simulink model "EOP_harness"  (Simulink 7.7)
settings: Solver=FixedStepDiscrete  SolverMode=SingleTasking  StartTime=0.0  StopTime=100  FixedStep=0.1  RelTol=1e-3
InitFcn:
  | CD_EOP_DEBOUNCE_OORH.DataType = 'uin16';
  | CD_EOP_DEBOUNCE_OORH = 10;
  | 
  | CD_EOP_DEBOUNCE_OORL.DataType = 'uin16';
  | CD_EOP_DEBOUNCE_OORL = 10;
  | 
  | 
  | 
  | if signalbuilder('EOP_harness/Signal_Builder','activegroup') == 1
  |   CD_EOP_FUNCTION.DataType = 'uint8';
  |   CD_EOP_FUNCTION.Value = 255;
  | elseif signalbuilder('EOP_harness/Signal_Builder','activegroup') == 7
  |   CD_EOP_FUNCTION.DataType = 'uint8';
  |   CD_EOP_FUNCTION.Value = 1;
  | elseif signalbuilder('EOP_harness/Signal_Builder','activegroup') == 8
  |   CD_EOP_FUNCTION.DataType = 'uint8';
  |   CD_EOP_FUNCTION.Value = 1;
  | elseif signalbuilder('EOP_harness/Signal_Builder','activegroup') == 3
  |   CD_EOP_FUNCTION.DataType = 'uint8';
  |   CD_EOP_FUNCTION.Value = 2;
  | else
  |   CD_EOP_FUNCTION.DataType = 'uint8';
  |   CD_EOP_FUNCTION.Value = 0;
  | end
  | 
  | 
  | if signalbuilder('EOP_harness/Signal_Builder','activegroup') == 4
  |   CD_EOP_FAULT_DETECTION_FUNCTION.DataType = 'uint8';
  |   CD_EOP_FAULT_DETECTION_FUNCTION.Value = 0;
  | end
  | 
  | if signalbuilder('EOP_harness/Signal_Builder','activegroup') == 5
  |   CD_SHUTDOWN_FUNCTION.DataType = 'uint8';
  |   CD_SHUTDOWN_FUNCTION.Value = 255;
  | elseif signalbuilder('EOP_harness/Signal_Builder','activegroup') == 8
  |   CD_SHUTDOWN_FUNCTION.DataType = 'uint8';
  |   CD_SHUTDOWN_FUNCTION.Value = 255;
  | else
  |   CD_SHUTDOWN_FUNCTION.DataType = 'uint8';
  |   CD_SHUTDOWN_FUNCTION.Value = 0;
  | end
  | 
  | if signalbuilder('EOP_harness/Signal_Builder','activegroup') == 12
  |   CD_ECU_FUNCTION.DataType = 'uint8';
  |   CD_ECU_FUNCTION.Value = 0;
  | else
  |   CD_ECU_FUNCTION.DataType = 'uint8';
  |   CD_ECU_FUNCTION.Value = 255;
  | end
undefined symbols (not defined in the file): CD_EOP_DEBOUNCE_EXTREMELY_LOW, CD_EOP_DEBOUNCE_NORMAL, CD_EOP_DEBOUNCE_SHUTDOWN, CD_EOP_FILTER_VALUE, CD_EOP_SWITCH_LOW, ENGINE_RUNNING, EXTREMELY_LOW, INIT_NORMAL, MXGTW_EOPGAUGE, MXGTW_EOPSHUTDOWN, MXGTW_EOPSND, MXGTW_EOPWARN, NON_FUNCTIONAL, NORMAL, SHUTDOWN, sigbuilder_block, srate100, SWITCH_INPUT
libraries: simulink x5, MX_Library x4
settings Model: Creator=spencermindeman  LastModifiedBy=aliebel  CovMetricSettings=dctw  CovModelRefEnable=off
settings MATStruct: SampleTime=0.01  Offset=0  Priority=[1.0]
settings DataIOCC: LimitDataPoints=off  SaveOutput=off  SaveTime=off
settings OptimizationCC: BlockReduction=off  InlineParams=on  ExpressionFolding=off  StateBitsets=on  DataBitsets=on  UseTempVars=on  InitFltsAndDblsToZero=on  NoFixptDivByZeroProtection=on  EfficientFloat2IntCast=on  OptimizeModelRefInitCode=on
settings DebuggingCC: SaveWithParameterizedLinksMsg=none  MultiTaskDSMMsg=warning  MultiTaskCondExecSysMsg=none  IntegerOverflowMsg=none  ModelReferenceCSMismatchMessage=warning
settings HardwareCC: ProdBitPerInt=16  ProdBitPerPointer=16  ProdIntDivRoundTo=Floor  ProdEndianess=BigEndian  ProdWordSize=16  ProdHWDeviceType=Motorola HC12
settings ModelReferenceCC: ModelReferenceNumInstancesAllowed=Single
settings RTWCC: SystemTargetFile=ert.tlc  GenCodeOnly=on  TemplateMakefile=ert_default_tmf  Description=Real-Time Workshop Embedded Coder (no auto configuration)  GenerateReport=on  RetainRTWFile=on  ProcessScript=ert_make_rtw_hook  IncludeHyperlinkInReport=on  LaunchReport=on  IncludeERTFirstTime=on
settings RTWCC: CustomHeaderCode=|
  | #include "cpp_req_defines.h"
  | #include "hw_fin.h"
  | #include "cdata.h"
settings CodeAppCC: IgnoreCustomStorageClasses=off  DefineNamingRule=UpperCase
settings ERTTargetCC: TargetFcnLib=ansi_tfl_tmw.mat  FunctionExecutionProfile=off  MultiwordLength=2048  GenerateSampleERTMain=on  IncludeMdlTerminateFcn=off  SupportAbsoluteTime=off  SupportNonFinite=off  SupportComplex=off  PurelyIntegerCode=on  ERTCustomFileTemplate=gen_rtw_req_defines_h.tlc  GlobalDataDefinition=InSeparateSourceFile  GlobalDataReference=InSeparateHeaderFile  ConvertIfToSwitch=off

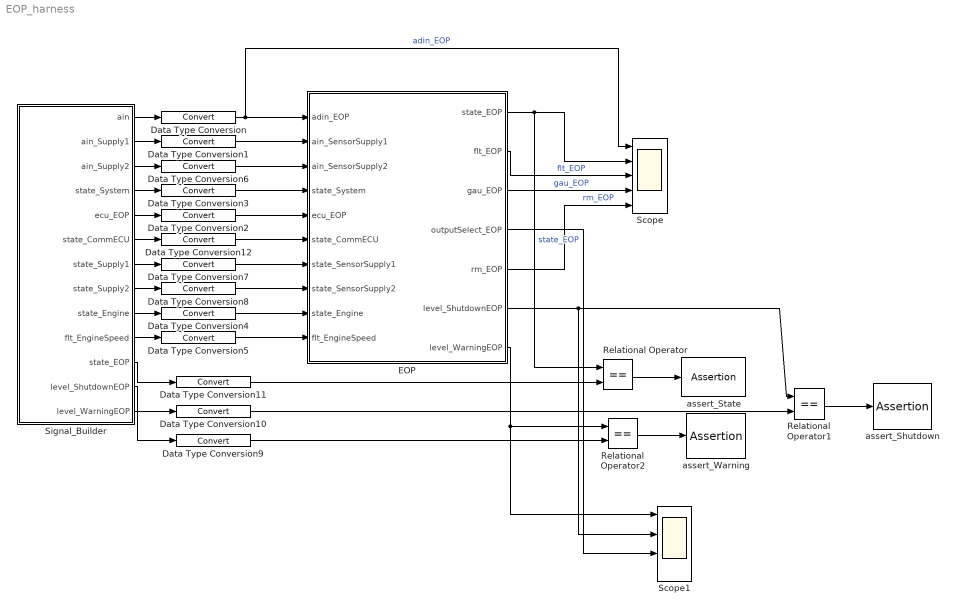
== system EOP_harness ==
  Data Type Conversion{,1..12} (13 alike) : DataTypeConversion
  EOP : Subsystem  TreatAsAtomicUnit=on  SystemSampleTime=srate100  RTWFileName=mod_Inputs
      settings: RTWSystemCode=Function  RTWFcnNameOpts=Use subsystem name  RTWFileNameOpts=User specified
  Relational Operator : RelationalOperator  Operator===  OutDataTypeStr=boolean
  Relational Operator1 : RelationalOperator  Operator===  OutDataTypeStr=boolean
  Relational Operator2 : RelationalOperator  Operator===  OutDataTypeStr=boolean
  Scope : Scope  NumInputPorts=5
      settings: TimeRange=6.671501087744744  YMin=130~8~10~2~160  YMax=210~14~30~4~250  MaxDataPoints=50000
  Scope1 : Scope  NumInputPorts=4
      settings: TimeRange=100  YMin=19.95~15.2~-1~-1  YMax=22.05~16.8~1~1  MaxDataPoints=50000
  Signal_Builder : Subsystem  Tag=STV Subsys  LoadFcn=sigbuilder_block('load');  StartFcn=sigbuilder_block('start');  StopFcn=sigbuilder_block('stop');  ClipboardFcn=sigbuilder_block('clipboard');  mask(Sigbuilder block){}
      mask help: Sigbuilder GUI
      mask init:
      | if ~strcmp(get_param(bdroot(gcbh),'SimulationStatus'),'stopped') tuvar = sigbuilder_block('maskInit'); end
      settings: CopyFcn=sigbuilder_block('copy');  DeleteFcn=sigbuilder_block('delete');  ModelCloseFcn=sigbuilder_block('modelClose');  PreSaveFcn=sigbuilder_block('preSave');  NameChangeFcn=sigbuilder_block('namechange');  OpenFcn=sigbuilder_block('open',[68.25 108 834.75 704.25 ]);  CloseFcn=sigbuilder_block('close');
      mask Display: plot(0,0,100,100,[10,10,40,40,10],[80,20,20,80,80],[40,10],[50,50], [40,27,10],[65,72,56],[40,25,25,10],[28,28,43,43]);
  assert_Shutdown : Assertion  Enabled=off
  assert_State : Assertion  Enabled=off
  assert_Warning : Assertion  Enabled=off
  wires:
  Signal_Builder/1(ain) -> Data Type Conversion/1
  Signal_Builder/2(ain_Supply1) -> Data Type Conversion1/1
  Signal_Builder/3(ain_Supply2) -> Data Type Conversion6/1
  Signal_Builder/4(state_System) -> Data Type Conversion3/1
  Signal_Builder/5(ecu_EOP) -> Data Type Conversion2/1
  Signal_Builder/7(state_Supply1) -> Data Type Conversion7/1
  Signal_Builder/8(state_Supply2) -> Data Type Conversion8/1
  Signal_Builder/9(state_Engine) -> Data Type Conversion4/1
  Signal_Builder/10(flt_EngineSpeed) -> Data Type Conversion5/1
  Data Type Conversion/1 -> Scope/1, EOP/1(adin_EOP)  "adin_EOP"
  Data Type Conversion1/1 -> EOP/2(ain_SensorSupply1)
  Data Type Conversion6/1 -> EOP/3(ain_SensorSupply2)
  Data Type Conversion3/1 -> EOP/4(state_System)
  Data Type Conversion7/1 -> EOP/7(state_SensorSupply1)
  Data Type Conversion8/1 -> EOP/8(state_SensorSupply2)
  Data Type Conversion4/1 -> EOP/9(state_Engine)
  Data Type Conversion5/1 -> EOP/10(flt_EngineSpeed)
  EOP/1(state_EOP) -> Relational Operator/1, Scope/2  "state_EOP"
  EOP/2(flt_EOP) -> Scope/3  "flt_EOP"
  EOP/3(gau_EOP) -> Scope/4  "gau_EOP"
  Data Type Conversion2/1 -> EOP/5(ecu_EOP)
  EOP/5(rm_EOP) -> Scope/5  "rm_EOP"
  Relational Operator/1 -> assert_State/1
  Signal_Builder/11(state_EOP) -> Data Type Conversion11/1
  Relational Operator1/1 -> assert_Shutdown/1
  Signal_Builder/12(level_ShutdownEOP) -> Data Type Conversion10/1
  EOP/6(level_ShutdownEOP) -> Relational Operator1/1, Scope1/2
  Relational Operator2/1 -> assert_Warning/1
  Signal_Builder/13(level_WarningEOP) -> Data Type Conversion9/1
  EOP/7(level_WarningEOP) -> Relational Operator2/1, Scope1/1
  Data Type Conversion9/1 -> Relational Operator2/2
  Data Type Conversion10/1 -> Relational Operator1/2
  Data Type Conversion11/1 -> Relational Operator/2
  EOP/4(outputSelect_EOP) -> Scope1/3
  Signal_Builder/6(state_CommECU) -> Data Type Conversion12/1
  Data Type Conversion12/1 -> EOP/6(state_CommECU)

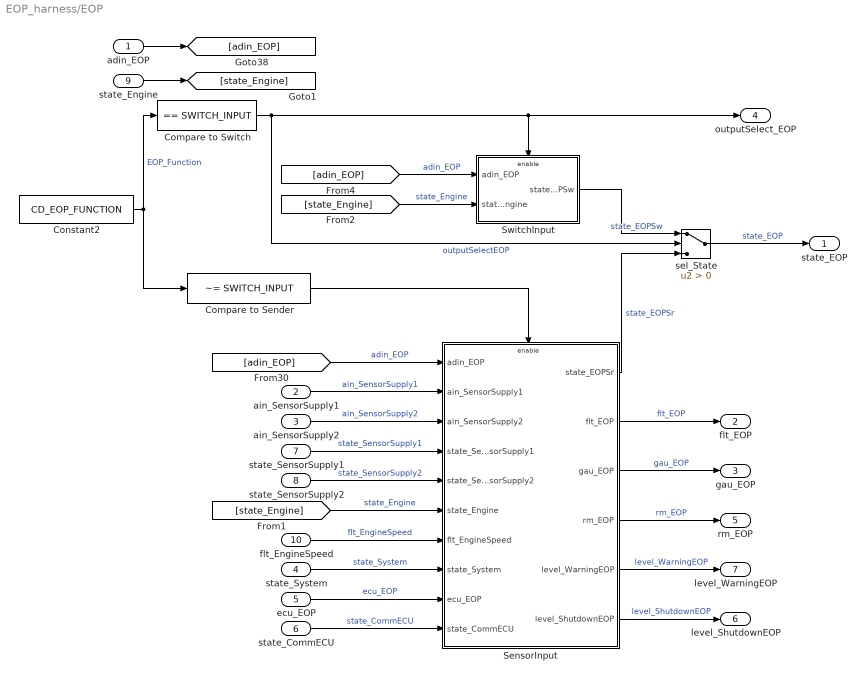
== system EOP_harness/EOP ==
  adin_EOP : Inport  OutDataTypeStr=uint16
  ain_SensorSupply1 : Inport  Port=2  OutDataTypeStr=uint16
  ain_SensorSupply2 : Inport  Port=3  OutDataTypeStr=uint16
  state_System : Inport  Port=4
  ecu_EOP : Inport  Port=5
  state_CommECU : Inport  Port=6
  state_SensorSupply1 : Inport  Port=7  OutDataTypeStr=uint8
  state_SensorSupply2 : Inport  Port=8  OutDataTypeStr=uint8
  state_Engine : Inport  Port=9  OutDataTypeStr=uint8
  flt_EngineSpeed : Inport  Port=10  OutDataTypeStr=uint16
  Compare to Sender : simulink/Logic and Bit Operations/Compare To Constant  SystemSampleTime=-1  relop=~=  const=SWITCH_INPUT  LogicOutDataTypeMode=boolean  ZeroCross=off
  Compare to Switch : simulink/Logic and Bit Operations/Compare To Constant  SystemSampleTime=-1  relop===  const=SWITCH_INPUT  LogicOutDataTypeMode=boolean  ZeroCross=off
  Constant2 : Constant  Value=CD_EOP_FUNCTION  OutDataTypeStr=uint8
  SensorInput : Subsystem  TreatAsAtomicUnit=on
  SwitchInput : Subsystem  TreatAsAtomicUnit=on
  sel_State : Switch  Criteria=u2 > Threshold  ZeroCross=off
      settings: AttributesFormatString=<threshold=%<Threshold>>
  state_EOP : Outport  OutDataTypeStr=uint8
  flt_EOP : Outport  Port=2  OutDataTypeStr=uint16
  gau_EOP : Outport  Port=3
  outputSelect_EOP : Outport  Port=4
  rm_EOP : Outport  Port=5
  level_ShutdownEOP : Outport  Port=6
  level_WarningEOP : Outport  Port=7
  wires:
  SensorInput/4(rm_EOP) -> rm_EOP/1  "rm_EOP"
  Compare to Sender/1 -> SensorInput/Enable
  [adin_EOP] -> SwitchInput/1(adin_EOP)  "adin_EOP"
  sel_State/1 -> state_EOP/1  "state_EOP"
  SwitchInput/1(state_EOPSw) -> sel_State/1  "state_EOPSw"
  SensorInput/1(state_EOPSr) -> sel_State/3  "state_EOPSr"
  SensorInput/3(gau_EOP) -> gau_EOP/1  "gau_EOP"
  adin_EOP/1 -> [adin_EOP]
  Constant2/1 -> Compare to Switch/1, Compare to Sender/1  "EOP_Function"
  Compare to Switch/1 -> sel_State/2, SwitchInput/Enable, outputSelect_EOP/1  "outputSelectEOP"
  state_Engine/1 -> [state_Engine]
  [state_Engine] -> SwitchInput/2(state_Engine)  "state_Engine"
  SensorInput/5(level_WarningEOP) -> level_WarningEOP/1  "level_WarningEOP"
  SensorInput/6(level_ShutdownEOP) -> level_ShutdownEOP/1  "level_ShutdownEOP"
  SensorInput/2(flt_EOP) -> flt_EOP/1  "flt_EOP"
  [adin_EOP] -> SensorInput/1(adin_EOP)  "adin_EOP"
  ain_SensorSupply1/1 -> SensorInput/2(ain_SensorSupply1)  "ain_SensorSupply1"
  ain_SensorSupply2/1 -> SensorInput/3(ain_SensorSupply2)  "ain_SensorSupply2"
  state_SensorSupply1/1 -> SensorInput/4(state_SensorSupply1)  "state_SensorSupply1"
  state_SensorSupply2/1 -> SensorInput/5(state_SensorSupply2)  "state_SensorSupply2"
  [state_Engine] -> SensorInput/6(state_Engine)  "state_Engine"
  flt_EngineSpeed/1 -> SensorInput/7(flt_EngineSpeed)  "flt_EngineSpeed"
  state_System/1 -> SensorInput/8(state_System)  "state_System"
  ecu_EOP/1 -> SensorInput/9(ecu_EOP)  "ecu_EOP"
  state_CommECU/1 -> SensorInput/10(state_CommECU)  "state_CommECU"

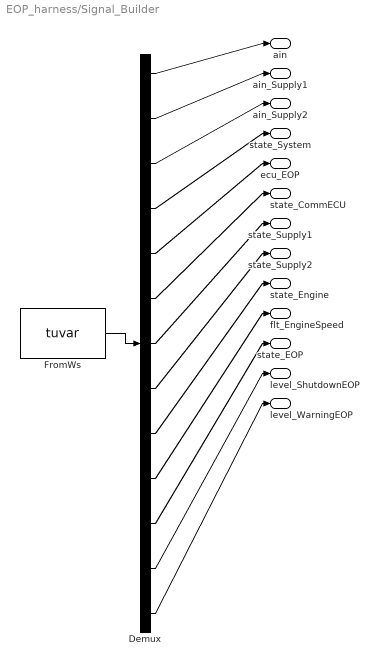
== system EOP_harness/Signal_Builder ==
  Demux : Demux  Tag=STV Demux  Outputs=13
  FromWs : FromWorkspace  Tag=STV FromWs  VariableName=tuvar  SampleTime=0  SigBuilderData=DataTag0  VnvData=DataTag1
  ain : Outport  Tag=STV Outport
  ain_Supply1 : Outport  Tag=STV Outport  Port=2
  ain_Supply2 : Outport  Tag=STV Outport  Port=3
  state_System : Outport  Tag=STV Outport  Port=4
  ecu_EOP : Outport  Tag=STV Outport  Port=5
  state_CommECU : Outport  Tag=STV Outport  Port=6
  state_Supply1 : Outport  Tag=STV Outport  Port=7
  state_Supply2 : Outport  Tag=STV Outport  Port=8
  state_Engine : Outport  Tag=STV Outport  Port=9
  flt_EngineSpeed : Outport  Tag=STV Outport  Port=10
  state_EOP : Outport  Tag=STV Outport  Port=11
  level_ShutdownEOP : Outport  Tag=STV Outport  Port=12
  level_WarningEOP : Outport  Tag=STV Outport  Port=13
  wires:
  FromWs/1 -> Demux/1
  Demux/1 -> ain/1
  Demux/2 -> ain_Supply1/1
  Demux/3 -> ain_Supply2/1
  Demux/4 -> state_System/1
  Demux/5 -> ecu_EOP/1
  Demux/6 -> state_CommECU/1
  Demux/7 -> state_Supply1/1
  Demux/8 -> state_Supply2/1
  Demux/9 -> state_Engine/1
  Demux/10 -> flt_EngineSpeed/1
  Demux/11 -> state_EOP/1
  Demux/12 -> level_ShutdownEOP/1
  Demux/13 -> level_WarningEOP/1

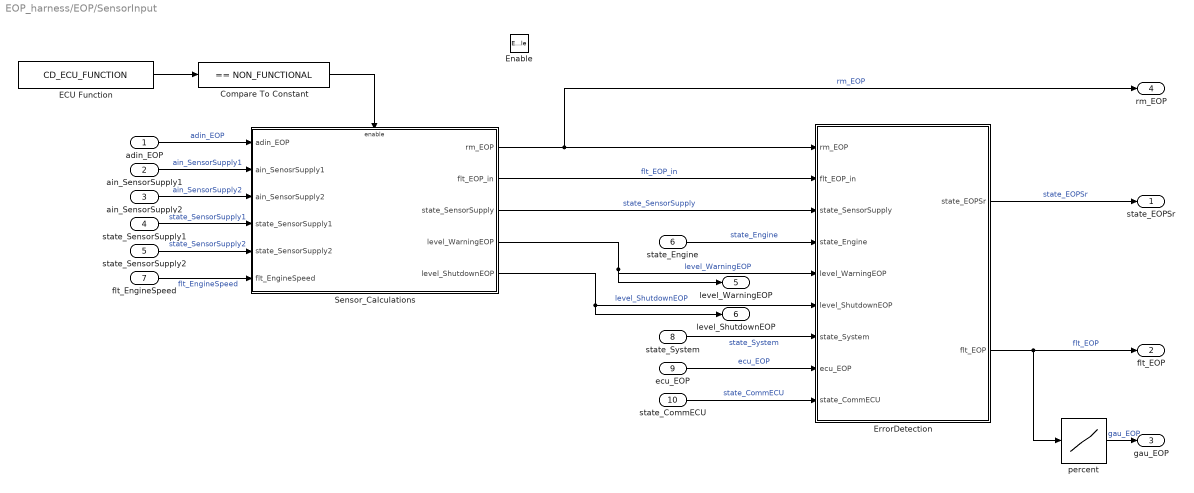
== system EOP_harness/EOP/SensorInput ==
  adin_EOP : Inport  OutDataTypeStr=uint16
  ain_SensorSupply1 : Inport  Port=2
  ain_SensorSupply2 : Inport  Port=3
  state_SensorSupply1 : Inport  Port=4  OutDataTypeStr=uint8
  state_SensorSupply2 : Inport  Port=5  OutDataTypeStr=uint8
  state_Engine : Inport  Port=6  OutDataTypeStr=uint8
  flt_EngineSpeed : Inport  Port=7
  state_System : Inport  Port=8
  ecu_EOP : Inport  Port=9  OutDataTypeStr=uint8
  state_CommECU : Inport  Port=10  OutDataTypeStr=uint8
  Enable : EnablePort  PropagateVarSize=During execution
      settings: AttributesFormatString=<states=%<StatesWhenEnabling>>
  Compare To Constant : simulink/Logic and Bit Operations/Compare To Constant  SystemSampleTime=-1  relop===  const=NON_FUNCTIONAL  LogicOutDataTypeMode=boolean  ZeroCross=off
  ECU Function : Constant  Value=CD_ECU_FUNCTION  OutDataTypeStr=uint8
  ErrorDetection : Stateflow chart  TreatAsAtomicUnit=on
  Sensor_Calculations : Subsystem  TreatAsAtomicUnit=on
  percent : Lookup  InputValues=[0:150]  Table=MXGTW_EOPGAUGE  LookUpMeth=Use Input Nearest  OutDataTypeStr=uint16  RndMeth=Zero  SaturateOnIntegerOverflow=on
      settings: AttributesFormatString=input = %<InputValues>\noutput = %<OutputValues>\nlookup = %<LookUpMeth>\nrounding = %<RndMeth>
  state_EOPSr : Outport  InitialOutput=[INIT_NORMAL]
  flt_EOP : Outport  Port=2  InitialOutput=[0]
  gau_EOP : Outport  Port=3  InitialOutput=[0]
  rm_EOP : Outport  Port=4  InitialOutput=[0]
  level_WarningEOP : Outport  Port=5  InitialOutput=[0]
  level_ShutdownEOP : Outport  Port=6  InitialOutput=[0]
  wires:
  state_System/1 -> ErrorDetection/7(state_System)  "state_System"
  percent/1 -> gau_EOP/1  "gau_EOP"
  state_Engine/1 -> ErrorDetection/4(state_Engine)  "state_Engine"
  Sensor_Calculations/3(state_SensorSupply) -> ErrorDetection/3(state_SensorSupply)  "state_SensorSupply"
  ErrorDetection/1(state_EOPSr) -> state_EOPSr/1  "state_EOPSr"
  ErrorDetection/2(flt_EOP) -> flt_EOP/1, percent/1  "flt_EOP"
  ecu_EOP/1 -> ErrorDetection/8(ecu_EOP)  "ecu_EOP"
  state_CommECU/1 -> ErrorDetection/9(state_CommECU)  "state_CommECU"
  adin_EOP/1 -> Sensor_Calculations/1(adin_EOP)  "adin_EOP"
  ain_SensorSupply1/1 -> Sensor_Calculations/2(ain_SenosrSupply1)  "ain_SensorSupply1"
  ain_SensorSupply2/1 -> Sensor_Calculations/3(ain_SensorSupply2)  "ain_SensorSupply2"
  state_SensorSupply1/1 -> Sensor_Calculations/4(state_SensorSupply1)  "state_SensorSupply1"
  state_SensorSupply2/1 -> Sensor_Calculations/5(state_SensorSupply2)  "state_SensorSupply2"
  flt_EngineSpeed/1 -> Sensor_Calculations/6(flt_EngineSpeed)  "flt_EngineSpeed"
  Sensor_Calculations/1(rm_EOP) -> ErrorDetection/1(rm_EOP), rm_EOP/1  "rm_EOP"
  Sensor_Calculations/2(flt_EOP_in) -> ErrorDetection/2(flt_EOP_in)  "flt_EOP_in"
  Sensor_Calculations/4(level_WarningEOP) -> ErrorDetection/5(level_WarningEOP), level_WarningEOP/1  "level_WarningEOP"
  Sensor_Calculations/5(level_ShutdownEOP) -> ErrorDetection/6(level_ShutdownEOP), level_ShutdownEOP/1  "level_ShutdownEOP"
  ECU Function/1 -> Compare To Constant/1
  Compare To Constant/1 -> Sensor_Calculations/Enable

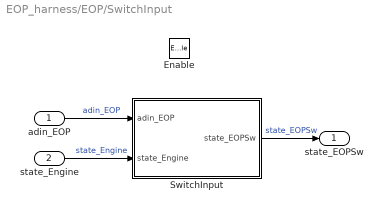
== system EOP_harness/EOP/SwitchInput ==
  adin_EOP : Inport
  state_Engine : Inport  Port=2
  Enable : EnablePort  PropagateVarSize=During execution
      settings: AttributesFormatString=<states=%<StatesWhenEnabling>>
  SwitchInput : Stateflow chart  TreatAsAtomicUnit=on
  state_EOPSw : Outport  InitialOutput=[INIT_NORMAL]
  wires:
  SwitchInput/1(state_EOPSw) -> state_EOPSw/1  "state_EOPSw"
  adin_EOP/1 -> SwitchInput/1(adin_EOP)  "adin_EOP"
  state_Engine/1 -> SwitchInput/2(state_Engine)  "state_Engine"

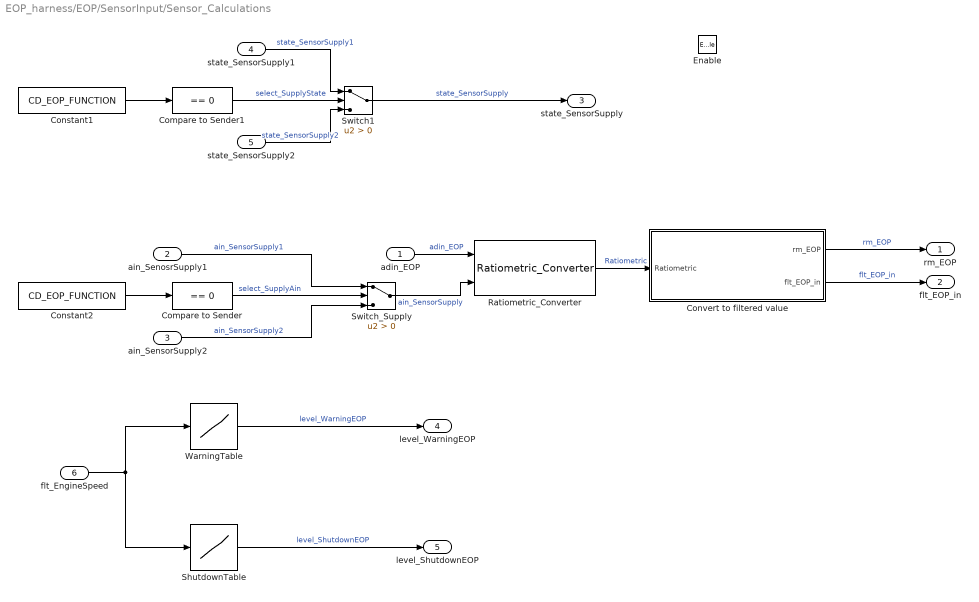
== system EOP_harness/EOP/SensorInput/Sensor_Calculations ==
  adin_EOP : Inport  OutDataTypeStr=uint16
  ain_SenosrSupply1 : Inport  Port=2  OutDataTypeStr=uint16
  ain_SensorSupply2 : Inport  Port=3  OutDataTypeStr=uint16
  state_SensorSupply1 : Inport  Port=4  OutDataTypeStr=uint8
  state_SensorSupply2 : Inport  Port=5  OutDataTypeStr=uint8
  flt_EngineSpeed : Inport  Port=6  OutDataTypeStr=uint16
  Enable : EnablePort  StatesWhenEnabling=reset  PropagateVarSize=During execution
      settings: AttributesFormatString=<states=%<StatesWhenEnabling>>
  Compare to Sender : simulink/Logic and Bit Operations/Compare To Constant  SystemSampleTime=-1  relop===  const=0  LogicOutDataTypeMode=boolean  ZeroCross=off
  Compare to Sender1 : simulink/Logic and Bit Operations/Compare To Constant  SystemSampleTime=-1  relop===  const=0  LogicOutDataTypeMode=boolean  ZeroCross=off
  Constant1 : Constant  Value=CD_EOP_FUNCTION  OutDataTypeStr=uint8
  Constant2 : Constant  Value=CD_EOP_FUNCTION  OutDataTypeStr=uint8
  Convert to filtered value : Subsystem
  Ratiometric_Converter : MX_Library/Ratiometric_Converter  SystemSampleTime=-1  multiplier=1000
  ShutdownTable : Lookup  InputValues=[0:100:5000]  Table=MXGTW_EOPSHUTDOWN  LookUpMeth=Use Input Nearest  OutDataTypeStr=uint16  RndMeth=Zero  SaturateOnIntegerOverflow=on
      settings: AttributesFormatString=input = %<InputValues>\noutput = %<OutputValues>\nlookup = %<LookUpMeth>\nrounding = %<RndMeth>
  Switch1 : Switch  Criteria=u2 > Threshold
  Switch_Supply : Switch  Criteria=u2 > Threshold
  WarningTable : Lookup  InputValues=[0:100:5000]  Table=MXGTW_EOPWARN  LookUpMeth=Use Input Nearest  OutDataTypeStr=uint16  RndMeth=Zero  SaturateOnIntegerOverflow=on
      settings: AttributesFormatString=input = %<InputValues>\noutput = %<OutputValues>\nlookup = %<LookUpMeth>\nrounding = %<RndMeth>
  rm_EOP : Outport  InitialOutput=[0]
  flt_EOP_in : Outport  Port=2  InitialOutput=[0]
  state_SensorSupply : Outport  Port=3  InitialOutput=[INIT_NORMAL]
  level_WarningEOP : Outport  Port=4  InitialOutput=[0]
  level_ShutdownEOP : Outport  Port=5  InitialOutput=[0]
  wires:
  Switch1/1 -> state_SensorSupply/1  "state_SensorSupply"
  state_SensorSupply2/1 -> Switch1/3  "state_SensorSupply2"
  Compare to Sender1/1 -> Switch1/2  "select_SupplyState"
  state_SensorSupply1/1 -> Switch1/1  "state_SensorSupply1"
  Constant1/1 -> Compare to Sender1/1
  Compare to Sender/1 -> Switch_Supply/2  "select_SupplyAin"
  Constant2/1 -> Compare to Sender/1
  Switch_Supply/1 -> Ratiometric_Converter/2  "ain_SensorSupply"
  ain_SensorSupply2/1 -> Switch_Supply/3  "ain_SensorSupply2"
  ain_SenosrSupply1/1 -> Switch_Supply/1  "ain_SensorSupply1"
  Convert to filtered value/1(rm_EOP) -> rm_EOP/1  "rm_EOP"
  adin_EOP/1 -> Ratiometric_Converter/1  "adin_EOP"
  WarningTable/1 -> level_WarningEOP/1  "level_WarningEOP"
  ShutdownTable/1 -> level_ShutdownEOP/1  "level_ShutdownEOP"
  flt_EngineSpeed/1 -> ShutdownTable/1, WarningTable/1
  Ratiometric_Converter/1 -> Convert to filtered value/1(Ratiometric)  "Ratiometric"
  Convert to filtered value/2(flt_EOP_in) -> flt_EOP_in/1  "flt_EOP_in"

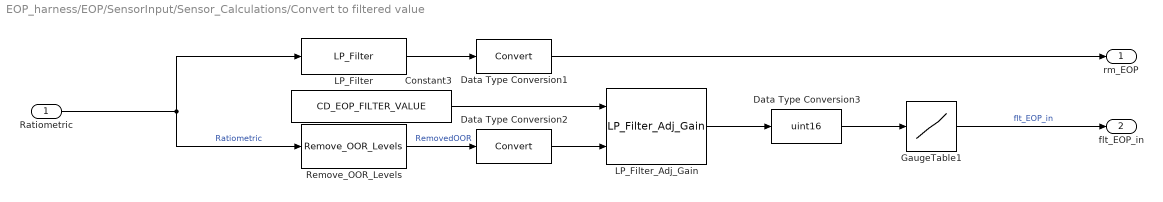
== system EOP_harness/EOP/SensorInput/Sensor_Calculations/Convert to filtered value ==
  Ratiometric : Inport
  Constant3 : Constant  Value=CD_EOP_FILTER_VALUE  OutDataTypeStr=uint8
  Data Type Conversion1 : DataTypeConversion
  Data Type Conversion2 : DataTypeConversion
  Data Type Conversion3 : DataTypeConversion  OutDataTypeStr=uint16
  GaugeTable1 : Lookup  InputValues=MXGTW_EOPSND  Table=[0:1:150]  LookUpMeth=Use Input Nearest  OutDataTypeStr=uint16  RndMeth=Zero  SaturateOnIntegerOverflow=on
      settings: AttributesFormatString=input = %<InputValues>\noutput = %<OutputValues>\nlookup = %<LookUpMeth>\nrounding = %<RndMeth>
  LP_Filter : MX_Library/LP_Filter  SystemSampleTime=-1  GAIN=3
  LP_Filter_Adj_Gain : MX_Library/LP_Filter_Adj_Gain  SystemSampleTime=-1
  Remove_OOR_Levels : MX_Library/Remove_OOR_Levels  SystemSampleTime=-1  OORL_LEVEL=CD_EOP_OORL  OORH_LEVEL=CD_EOP_OORH
  rm_EOP : Outport
  flt_EOP_in : Outport  Port=2
  wires:
  Constant3/1 -> LP_Filter_Adj_Gain/1
  LP_Filter/1 -> Data Type Conversion1/1
  Data Type Conversion3/1 -> GaugeTable1/1
  LP_Filter_Adj_Gain/1 -> Data Type Conversion3/1
  Data Type Conversion2/1 -> LP_Filter_Adj_Gain/2
  Remove_OOR_Levels/1 -> Data Type Conversion2/1  "RemovedOOR"
  Ratiometric/1 -> Remove_OOR_Levels/1, LP_Filter/1  "Ratiometric"
  Data Type Conversion1/1 -> rm_EOP/1
  GaugeTable1/1 -> flt_EOP_in/1  "flt_EOP_in"

== stateflow chart EOP/SensorInput/ErrorDetection ==
  state SENSOR
    state STATE [parallel]
      settings: executionOrder=2
      state NON_FUNCTIONAL
        en:state_EOPSr = NORMAL;
      state NORMAL
        state NORMAL
          state NORMAL
            state_EOPSr = NORMAL;
          state DEBOUNCE
            en:debounceCount = 0;
            du:debounceCount++;
          SENSOR.STATE.NORMAL.NORMAL.DEBOUNCE -> SENSOR.STATE.NORMAL.NORMAL.NORMAL : [(debounceCount >= CD_EOP_DEBOUNCE_NORMAL)...
              | || (state_EOPSr == NORMAL)]
          (default) -> SENSOR.STATE.NORMAL.NORMAL.DEBOUNCE
        state EXTREMELY_LOW
          state EXTREMELY_LOW
            state_EOPSr = EXTREMELY_LOW;
          state DEBOUNCE
            en:debounceCount = 0;
            du:debounceCount++;
          SENSOR.STATE.NORMAL.EXTREMELY_LOW.DEBOUNCE -> SENSOR.STATE.NORMAL.EXTREMELY_LOW.EXTREMELY_LOW : [(debounceCount >= CD_EOP_DEBOUNCE_EXTREMELY_LOW)...
              | || (state_EOPSr == EXTREMELY_LOW)]
          (default) -> SENSOR.STATE.NORMAL.EXTREMELY_LOW.DEBOUNCE
        state LOW
          state LOW
            state_EOPSr = LOW;
          state DEBOUNCE
            en:debounceCount = 0;
            du:debounceCount++;
          SENSOR.STATE.NORMAL.LOW.DEBOUNCE -> SENSOR.STATE.NORMAL.LOW.LOW : [(debounceCount >= CD_EOP_DEBOUNCE_LOW)...
              | || (state_EOPSr == LOW)]
          (default) -> SENSOR.STATE.NORMAL.LOW.DEBOUNCE
        state SHUTDOWN
          state SHUTDOWN
            state_EOPSr = SHUTDOWN;
          state DEBOUNCE
            en:debounceCount = 0;
            du:debounceCount++;
          SENSOR.STATE.NORMAL.SHUTDOWN.DEBOUNCE -> SENSOR.STATE.NORMAL.SHUTDOWN.SHUTDOWN : [(debounceCount >= CD_EOP_DEBOUNCE_SHUTDOWN)]
          (default) -> SENSOR.STATE.NORMAL.SHUTDOWN.DEBOUNCE
        SENSOR.STATE.NORMAL.SHUTDOWN -> SENSOR.STATE.NORMAL.LOW : [(flt_EOP_in > (level_ShutdownEOP + CD_PRESSURE_HYSTERESIS))...
            | && (state_EOPSr != SHUTDOWN)]
        SENSOR.STATE.NORMAL.EXTREMELY_LOW -> SENSOR.STATE.NORMAL.SHUTDOWN [order 2] : [(CD_SHUTDOWN_FUNCTION != NON_FUNCTIONAL)...
            | && (state_EOPSr == EXTREMELY_LOW)]
        SENSOR.STATE.NORMAL.EXTREMELY_LOW -> SENSOR.STATE.NORMAL.LOW [order 1] : [(flt_EOP_in > (level_ShutdownEOP + CD_PRESSURE_HYSTERESIS))...
            | && (flt_EOP_in <= level_WarningEOP)]
        SENSOR.STATE.NORMAL.LOW -> SENSOR.STATE.NORMAL.EXTREMELY_LOW [order 2] : [(flt_EOP_in <= level_ShutdownEOP)]
        SENSOR.STATE.NORMAL.NORMAL -> SENSOR.STATE.NORMAL.LOW [order 1] : [(flt_EOP_in <= level_WarningEOP)...
            | && (flt_EOP_in > level_ShutdownEOP) ...
            | && (state_Engine == ENGINE_RUNNING)...
            | && (CD_EOP_FAULT_DETECTION_FUNCTION != NON_FUNCTIONAL)]
        SENSOR.STATE.NORMAL.LOW -> SENSOR.STATE.NORMAL.NORMAL [order 1] : [(flt_EOP_in > (level_WarningEOP + CD_PRESSURE_HYSTERESIS))...
            | || (state_Engine != ENGINE_RUNNING)]
        SENSOR.STATE.NORMAL.EXTREMELY_LOW -> SENSOR.STATE.NORMAL.NORMAL [order 3] : [(flt_EOP_in > (level_WarningEOP + CD_PRESSURE_HYSTERESIS))...
            | || (state_Engine != ENGINE_RUNNING)]
        SENSOR.STATE.NORMAL.NORMAL -> SENSOR.STATE.NORMAL.EXTREMELY_LOW [order 2] : [(flt_EOP_in <= level_ShutdownEOP)...
            | && (state_Engine == ENGINE_RUNNING)...
            | && (CD_EOP_FAULT_DETECTION_FUNCTION != NON_FUNCTIONAL)]
        (default) -> SENSOR.STATE.NORMAL.NORMAL
      state OUT_OF_RANGE_HIGH
        state OORH
          state_EOPSr = OORH;
        state DEBOUNCE
          en:debounceCount = 0;
          du:debounceCount++;
        SENSOR.STATE.OUT_OF_RANGE_HIGH.DEBOUNCE -> OORH : [(debounceCount >= CD_EOP_DEBOUNCE_OORH)...
            | || (state_EOPSr == OORH)]
        (default) -> SENSOR.STATE.OUT_OF_RANGE_HIGH.DEBOUNCE
      state OUT_OF_RANGE_LOW
        state OORL
          state_EOPSr = OORL;
        state DEBOUNCE
          en:debounceCount = 0;
          du:debounceCount++;
        SENSOR.STATE.OUT_OF_RANGE_LOW.DEBOUNCE -> OORL : [(debounceCount >= CD_EOP_DEBOUNCE_OORL)...
            | || (state_EOPSr == OORL)]
        (default) -> SENSOR.STATE.OUT_OF_RANGE_LOW.DEBOUNCE
      (default) -> NON_FUNCTIONAL
      SENSOR.STATE.NORMAL -> NON_FUNCTIONAL [order 1] : [(state_SensorSupply != NORMAL)...
          | || (state_System != SYS_NORMAL)]
      NON_FUNCTIONAL -> SENSOR.STATE.NORMAL : [(CD_EOP_FUNCTION != NON_FUNCTIONAL)...
          | && (state_SensorSupply == NORMAL)...
          | && (state_System == SYS_NORMAL)]
      SENSOR.STATE.NORMAL -> OUT_OF_RANGE_HIGH [order 3] : [(rm_EOP >= CD_EOP_OORH)...
          | && (state_EOPSr != SHUTDOWN)]
      OUT_OF_RANGE_HIGH -> SENSOR.STATE.NORMAL [order 1] : [(rm_EOP < CD_EOP_OORH)]
      SENSOR.STATE.NORMAL -> OUT_OF_RANGE_LOW [order 2] : [(rm_EOP <= CD_EOP_OORL)...
          | && (state_EOPSr != SHUTDOWN)]
      OUT_OF_RANGE_LOW -> SENSOR.STATE.NORMAL [order 1] : [(rm_EOP > CD_EOP_OORL)]
      OUT_OF_RANGE_HIGH -> NON_FUNCTIONAL [order 2] : [(state_SensorSupply != NORMAL)...
          | && (state_EOPSr != OORH)]
      OUT_OF_RANGE_LOW -> NON_FUNCTIONAL [order 2] : [(state_SensorSupply != NORMAL)...
          | && (state_EOPSr != OORL)]
    state VALUE [parallel]
      settings: executionOrder=1
      state INIT
        en:flt_EOP = 0;
        (default) -> (junction 31)
        (junction 31) -> (junction 32) [order 1] : [((rm_EOP <= CD_EOP_OORL) || (rm_EOP >= CD_EOP_OORH))]
        (junction 31) -> (junction 33) [order 2] : {
            | flt_EOP = flt_EOP_in;
            | }
        (junction 32) -> (junction 34) : {
            | flt_EOP = 0;
            | }
        (junction 34) -> (junction 33)
      state NORMAL
        du:flt_EOP = flt_EOP_in;
      (default) -> INIT
      INIT -> SENSOR.VALUE.NORMAL : [(state_System == SYS_NORMAL)]
  state ECU
    state NORMAL
      en:state_EOPSr = NORMAL;
      du:flt_EOP = ecu_EOP;
    state NO_COMMUNICATION
      en:flt_EOP = 0;
    (default) -> ECU.NORMAL
    ECU.NORMAL -> NO_COMMUNICATION : [(state_CommECU == NO_COMMUNICATION)]
    NO_COMMUNICATION -> ECU.NORMAL : [(state_CommECU != NO_COMMUNICATION)]
  (default) -> SENSOR
  SENSOR -> ECU : [(CD_ECU_FUNCTION != NON_FUNCTIONAL)]
  data: rm_EOP input uint16; flt_EOP_in input uint16; state_EOPSr output uint8; state_SensorSupply input double; state_Engine input double; CD_EOP_FUNCTION parameter uint8; CD_EOP_OORH parameter uint16; CD_EOP_OORL parameter uint16; CD_EOP_DEBOUNCE_OORH parameter uint16; CD_EOP_DEBOUNCE_OORL parameter uint16; CD_EOP_DEBOUNCE_NORMAL parameter uint16; CD_EOP_DEBOUNCE_LOW parameter uint16; CD_EOP_DEBOUNCE_EXTREMELY_LOW parameter uint16; CD_EOP_DEBOUNCE_SHUTDOWN parameter uint16; debounceCount local uint16 =0; level_WarningEOP input uint16; level_ShutdownEOP input uint16; CD_SHUTDOWN_FUNCTION parameter uint8; CD_PRESSURE_HYSTERESIS parameter uint16; ENGINE_RUNNING parameter uint8 =3; EXTREMELY_LOW parameter uint8 =14; LOW parameter uint8 =9; NORMAL parameter uint8 =8; OORH parameter uint8 =21; OORL parameter uint8 =22; SHUTDOWN parameter uint8 =15; NON_FUNCTIONAL parameter uint8 =8; state_System input uint8; SYS_NORMAL parameter uint8; flt_EOP output uint16; CD_ECU_FUNCTION parameter uint8; ecu_EOP input uint8; state_CommECU input uint8; NO_COMMUNICATION parameter uint8; CD_EOP_FAULT_DETECTION_FUNCTION parameter uint8

== stateflow chart EOP/SwitchInput/SwitchInput ==
  state SHUTDOWN
    state SHUTDOWN
      en:state_EOPSw = SHUTDOWN;
    state DEBOUNCE
      en:debounceCount = 0;
      du:debounceCount++;
    DEBOUNCE -> SHUTDOWN.SHUTDOWN : [(debounceCount >= CD_EOP_DEBOUNCE_SHUTDOWN)]
    (default) -> DEBOUNCE
  state EXTREMELY_LOW
    state EXTREMELY_LOW
      en:state_EOPSw = EXTREMELY_LOW;
    state DEBOUNCE_EXTREMELY_LOW
      en:debounceCount = 0;
      du:debounceCount++;
    (default) -> DEBOUNCE_EXTREMELY_LOW
    DEBOUNCE_EXTREMELY_LOW -> EXTREMELY_LOW.EXTREMELY_LOW : [(debounceCount >= CD_EOP_DEBOUNCE_EXTREMELY_LOW)...
        | || (state_EOPSw == EXTREMELY_LOW)]
  state NORMAL
    state NORMAL
      en:state_EOPSw = NORMAL;
    state DEBOUNCE_NORMAL
      en:debounceCount = 0;
      du:debounceCount++;
    (default) -> DEBOUNCE_NORMAL
    DEBOUNCE_NORMAL -> NORMAL.NORMAL : [(debounceCount >= CD_EOP_DEBOUNCE_NORMAL)...
        | || (state_EOPSw == NORMAL)]
  NORMAL -> EXTREMELY_LOW : [(adin_EOP <= CD_EOP_SWITCH_LOW)...
      | && (state_Engine == ENGINE_RUNNING)]
  EXTREMELY_LOW -> NORMAL [order 1] : [(adin_EOP >= CD_EOP_SWITCH_LOW)...
      | || (state_Engine != ENGINE_RUNNING)]
  SHUTDOWN -> EXTREMELY_LOW : [((adin_EOP >= CD_EOP_SWITCH_LOW) || (state_Engine != ENGINE_RUNNING))...
      | && (state_EOPSw != SHUTDOWN)]
  EXTREMELY_LOW -> SHUTDOWN [order 2] : [(CD_SHUTDOWN_FUNCTION != NON_FUNCTIONAL)...
      | && (state_EOPSw == EXTREMELY_LOW)]
  (default) -> NORMAL.NORMAL
  data: adin_EOP input uint16; state_EOPSw output uint8; debounceCount local uint16 =0; CD_EOP_DEBOUNCE_NORMAL parameter uint16; CD_EOP_DEBOUNCE_SHUTDOWN parameter uint16; state_Engine input uint8; CD_SHUTDOWN_FUNCTION parameter uint8; ENGINE_RUNNING parameter uint8 =3; NORMAL parameter uint8 =8; SHUTDOWN parameter uint8 =15; CD_EOP_SWITCH_LOW parameter uint16; NON_FUNCTIONAL parameter uint8 =8; EXTREMELY_LOW parameter uint8 =14; CD_EOP_DEBOUNCE_EXTREMELY_LOW parameter uint16
